simulink model "mixing_diode_model_2022b"  (R2022b)
settings: Solver=ode45  StartTime=0.0  StopTime=10  RelTol=1e-3  EnableMultiTasking=on
libraries: dsparch4 x1
settings Model: Creator=morelos_zaragoza  LastModifiedBy=14083
settings SolverCC: AlgebraicLoopSolver=TrustRegion
settings DataIOCC: LimitDataPoints=on  SaveFormat=Array  SignalLoggingSaveFormat=ModelDataLogs  ReturnWorkspaceOutputs=off
settings OptimizationCC: ExpressionDepthLimit=2147483647  InitFltsAndDblsToZero=on  LifeSpan=inf
settings DebuggingCC: SaveWithParameterizedLinksMsg=none  UnderspecifiedInitializationDetection=Classic  MergeDetectMultiDrivingBlocksExec=none  SignalResolutionControl=TryResolveAllWithWarning  SolverPrmCheckMsg=warning  MultiTaskDSMMsg=warning  MultiTaskCondExecSysMsg=none  FcnCallInpInsideContextMsg=warning  UnconnectedInputMsg=warning  UnconnectedOutputMsg=warning  UnconnectedLineMsg=warning  StateNameClashWarn=warning  SFUnexpectedBacktrackingDiag=warning  SFNoUnconditionalDefaultTransitionDiag=warning  SFExecutionAtInitializationDiag=none  SFMachineParentedDataDiag=warning  ArithmeticOperatorsInVariantConditions=warning
settings HardwareCC: ProdBitPerPointer=32  ProdBitPerSizeT=32  ProdBitPerPtrDiffT=32  ProdLargestAtomicFloat=None  ProdIntDivRoundTo=Undefined  ProdEndianess=Unspecified  ProdWordSize=32  ProdHWDeviceType=32-bit Generic
settings ModelReferenceCC: PropagateSignalLabelsOutOfModel=off
settings SFSimCC: SimUseLocalCustomCode=off  CustomCodeUndefinedFunction=UseInterfaceOnly
settings RTWCC: RTWUseLocalCustomCode=off
settings CodeAppCC: StateflowObjectComments=on
settings GRTTargetCC: TargetFcnLib=ansi_tfl_tmw.mat  TargetLangStandard=C89/C90 (ANSI)  CombineOutputUpdateFcns=off  GRTInterface=on
settings ConfigComp: CovMetricSettings=dw  CovSaveCumulativeToWorkspaceVar=on  CovSaveSingleToWorkspaceVar=on  CovExternalEMLEnable=off

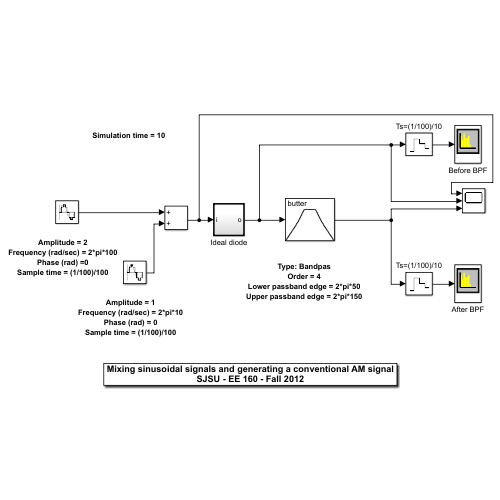
[thumbnail: Simulink's stored preview of the top-level diagram]
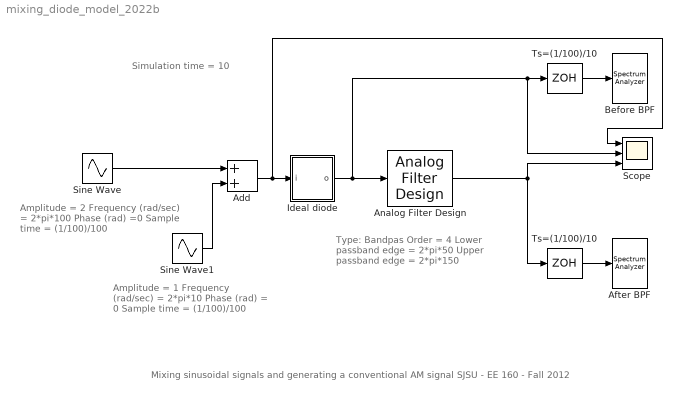
== system mixing_diode_model_2022b ==
  note: Amplitude = 2
      | Frequency (rad/sec) = 2*pi*100
      | Phase (rad) =0
      | Sample time = (1/100)/100
  note: Simulation time = 10
  note: Mixing sinusoidal signals and generating a conventional AM signal
      | SJSU - EE 160 - Fall 2012
  note: Amplitude = 1
      | Frequency (rad/sec) = 2*pi*10
      | Phase (rad) = 0
      | Sample time = (1/100)/100
  note: Type: Bandpas
      | Order = 4
      | Lower passband edge = 2*pi*50
      | Upper passband edge = 2*pi*150
  " Ts=(1/100)/10 " : ZeroOrderHold  SampleTime=(1/100)/10
  Add : Sum
  After BPF : SpectrumAnalyzer
  Analog Filter Design : dsparch4/Analog Filter Design  method=Butterworth  filttype=Bandpass  N=8  Wlo=2*pi*50  Whi=2*pi*150  Rp=2  Rs=40
  Before BPF : SpectrumAnalyzer
  Ideal diode : Subsystem  TreatAsAtomicUnit=on
  Scope : Scope  NumInputPorts=3
  Sine Wave : Sin  Amplitude=2  Frequency=2*pi*100  SampleTime=(1/100)/100
  Sine Wave1 : Sin  Frequency=2*pi*10  SampleTime=(1/100)/100
  Ts=(1/100)/10 : ZeroOrderHold  SampleTime=(1/100)/10
  wires:
  Add/1 -> Scope/1, Ideal diode/1(i)
  Sine Wave/1 -> Add/1
  Sine Wave1/1 -> Add/2
  Ideal diode/1(o) -> Analog Filter Design/1, Ts=(1/100)/10/1, Scope/2
  " Ts=(1/100)/10 "/1 -> After BPF/1
  Ts=(1/100)/10/1 -> Before BPF/1
  Analog Filter Design/1 -> Scope/3, " Ts=(1/100)/10 "/1

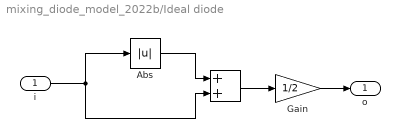
== system mixing_diode_model_2022b/Ideal diode ==
  i : Inport
  " " : Sum
  Abs : Abs  SaturateOnIntegerOverflow=off
  Gain : Gain  Gain=1/2
  o : Outport
  wires:
  i/1 -> Abs/1, " "/2
  Abs/1 -> " "/1
  " "/1 -> Gain/1
  Gain/1 -> o/1
